simulink model "simon_loop_unrolling_4"  (R2015b)
settings: Solver=FixedStepDiscrete  SolverMode=SingleTasking  StartTime=0.0  StopTime=5e-4  RelTol=1e-3
undefined symbols (not defined in the file): a, b
libraries: shlslibv1 x190
settings Model: synDspstartup=OK  Creator=pgali  LastModifiedBy=sjparekh
settings DataIOCC: SaveOutput=off  SignalLogging=off  SaveTime=off
settings OptimizationCC: DefaultParameterBehavior=Inlined
settings DebuggingCC: AlgebraicLoopMsg=error  InheritedTsInSrcMsg=none

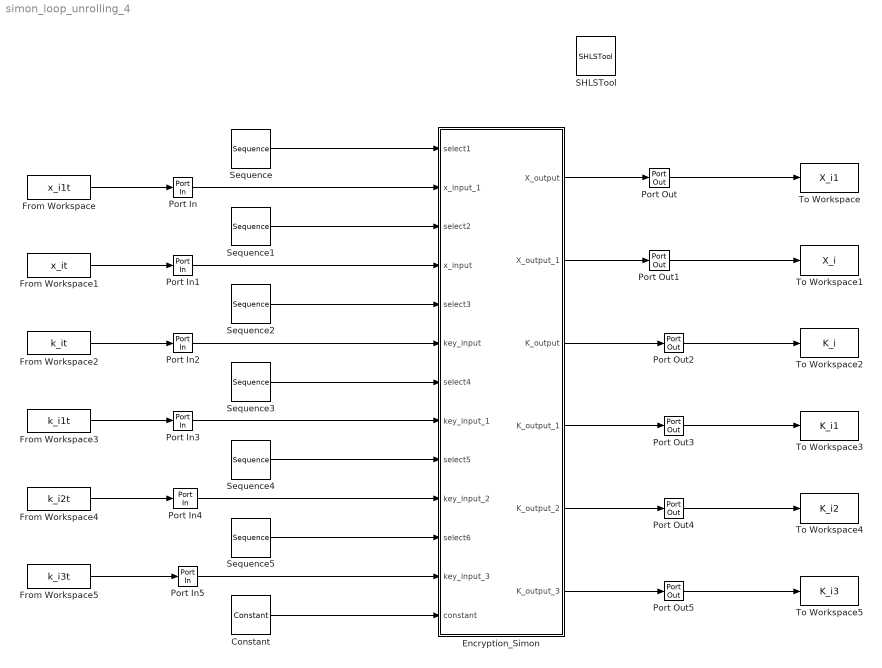
== system simon_loop_unrolling_4 ==
  Constant : shlslibv1/Sources/Constant  syn_cst_val=65532  syn_cst_format=Automatic  syn_cst_wl=1  syn_cst_fl=0  syn_cst_dt=unsigned  syn_cst_rnd=on  syn_cst_st=1/748e6  synBlockType=primitive  synLatency=0  synBlockId=15
  "Encryption_Simon " : Subsystem
  From Workspace : FromWorkspace  VariableName=x_i1t  SampleTime=0
  From Workspace1 : FromWorkspace  VariableName=x_it  SampleTime=0
  From Workspace2 : FromWorkspace  VariableName=k_it  SampleTime=0
  From Workspace3 : FromWorkspace  VariableName=k_i1t  SampleTime=0
  From Workspace4 : FromWorkspace  VariableName=k_i2t  SampleTime=0
  From Workspace5 : FromWorkspace  VariableName=k_i3t  SampleTime=0
  Port In{,1..5} (6 alike) : shlslibv1/Ports & Subsystems/Port In  syn_out_wl=16  syn_out_fl=0  syn_out_dt=unsigned  syn_out_st=1/748e6  syn_capture=off  syn_register=on  syn_out_sat=off  syn_out_rnd=on  synBlockType=port  synLatency=1  synBlockId=0
  Port Out{,1..5} (6 alike) : shlslibv1/Ports & Subsystems/Port Out  syn_capture=off  syn_register=on  synBlockType=port  synLatency=1  synBlockId=1
  SHLSTool : shlslibv1/SHLSTool  synBlockType=tool  syn_dsp_mode=FPGA
  Sequence{,1..5} (6 alike) : shlslibv1/Sources/Sequence  syn_seq_vec=[0 0 0 0 1 1 1 1 1 1 1 1 1 1 1 1 1 1 1 1 1 1 1 1 1 1 1 1 1 1 1 1]  syn_seq_wl=1  syn_seq_fl=0  syn_seq_dt=unsigned  syn_rst_port=off  syn_en_port=off  syn_seq_st=1/748e6  synBlockType=custom  synLatency=1
  To Workspace : ToWorkspace  VariableName=X_i1  SaveFormat=Structure With Time  SampleTime=-1
  To Workspace1 : ToWorkspace  VariableName=X_i  SaveFormat=Structure With Time  SampleTime=-1
  To Workspace2 : ToWorkspace  VariableName=K_i  SaveFormat=Structure With Time  SampleTime=-1
  To Workspace3 : ToWorkspace  VariableName=K_i1  SaveFormat=Structure With Time  SampleTime=-1
  To Workspace4 : ToWorkspace  VariableName=K_i2  SaveFormat=Structure With Time  SampleTime=-1
  To Workspace5 : ToWorkspace  VariableName=K_i3  SaveFormat=Structure With Time  SampleTime=-1
  wires:
  From Workspace1/1 -> Port In1/1
  From Workspace2/1 -> Port In2/1
  "Encryption_Simon "/1(X_output) -> Port Out/1
  "Encryption_Simon "/2(X_output_1) -> Port Out1/1
  "Encryption_Simon "/3(K_output) -> Port Out2/1
  "Encryption_Simon "/4(K_output_1) -> Port Out3/1
  "Encryption_Simon "/5(K_output_2) -> Port Out4/1
  "Encryption_Simon "/6(K_output_3) -> Port Out5/1
  From Workspace/1 -> Port In/1
  Constant/1 -> "Encryption_Simon "/13(constant)
  From Workspace3/1 -> Port In3/1
  From Workspace4/1 -> Port In4/1
  From Workspace5/1 -> Port In5/1
  Port In/1 -> "Encryption_Simon "/2(x_input_1)
  Port In1/1 -> "Encryption_Simon "/4(x_input)
  Port In2/1 -> "Encryption_Simon "/6(key_input)
  Port In3/1 -> "Encryption_Simon "/8(key_input_1)
  Port In4/1 -> "Encryption_Simon "/10(key_input_2)
  Port In5/1 -> "Encryption_Simon "/12(key_input_3)
  Port Out/1 -> To Workspace/1
  Port Out1/1 -> To Workspace1/1
  Port Out3/1 -> To Workspace3/1
  Port Out4/1 -> To Workspace4/1
  Port Out5/1 -> To Workspace5/1
  Port Out2/1 -> To Workspace2/1
  Sequence/1 -> "Encryption_Simon "/1(select1)
  Sequence1/1 -> "Encryption_Simon "/3(select2)
  Sequence2/1 -> "Encryption_Simon "/5(select3)
  Sequence3/1 -> "Encryption_Simon "/7(select4)
  Sequence4/1 -> "Encryption_Simon "/9(select5)
  Sequence5/1 -> "Encryption_Simon "/11(select6)

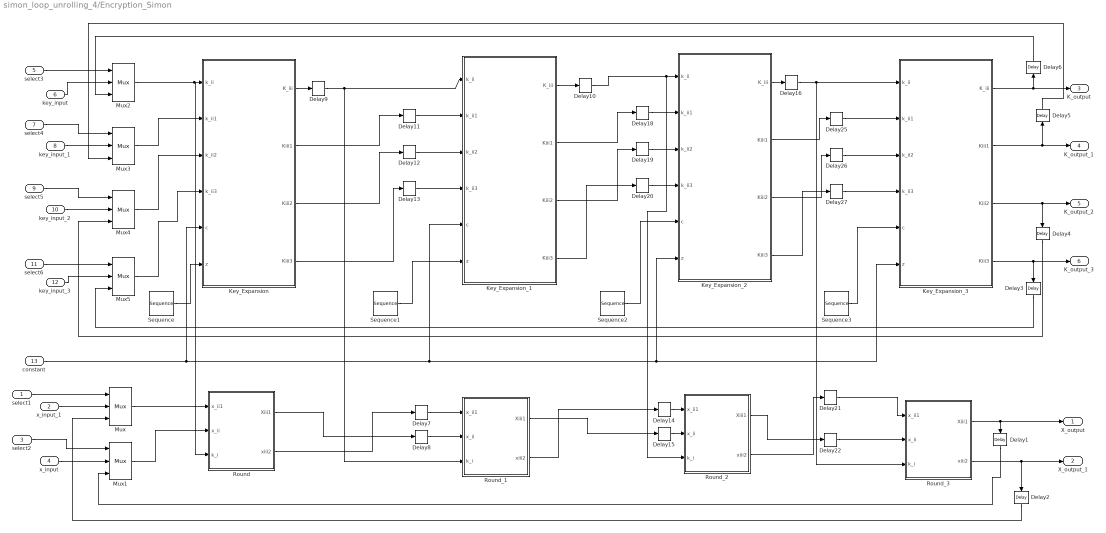
== system simon_loop_unrolling_4/Encryption_Simon  ==
  select1 : Inport
  x_input_1 : Inport  Port=2
  select2 : Inport  Port=3
  x_input : Inport  Port=4
  select3 : Inport  Port=5
  key_input : Inport  Port=6
  select4 : Inport  Port=7
  key_input_1 : Inport  Port=8
  select5 : Inport  Port=9
  key_input_2 : Inport  Port=10
  select6 : Inport  Port=11
  key_input_3 : Inport  Port=12
  constant : Inport  Port=13
  Delay{1..16,18..22,25..27} (24 alike) : shlslibv1/Memories/Delay  syn_delay_val=1  synBlockType=primitive  synLatency=1  synBlockId=104
  Key_Expansion : Subsystem
  Key_Expansion_1 : Subsystem
  Key_Expansion_2 : Subsystem
  Key_Expansion_3 : Subsystem
  Mux{,1..5} (6 alike) : shlslibv1/Signal Operations/Mux  syn_in_nb=2  syn_out_f=Full Precision  syn_out_wl=16  syn_out_fl=8  syn_out_dt=signed  syn_en_se=off  synBlockType=primitive  synLatency=0  synBlockId=16
  Round : Subsystem
  Round_1 : Subsystem
  Round_2 : Subsystem
  Round_3 : Subsystem
  Sequence : shlslibv1/Sources/Sequence  syn_seq_vec=[1 1 1 1 1 1 1 1 0 0 0 0 0 0 0 0 0 0 0 0 0 0 0 0 1 1 1 1 1 1 1 1]  syn_seq_wl=16  syn_seq_fl=0  syn_seq_dt=unsigned  syn_rst_port=off  syn_en_port=off  syn_seq_st=-1  synBlockType=custom  synLatency=1
  Sequence1 : shlslibv1/Sources/Sequence  syn_seq_vec=[0 1 1 1 1 0 0 0 0 0 0 0 0 1 1 1 1 1 1 1 1 0 0 0 0 1 1 1 1 1 1 1]  syn_seq_wl=16  syn_seq_fl=0  syn_seq_dt=unsigned  syn_rst_port=off  syn_en_port=off  syn_seq_st=-1  synBlockType=custom  synLatency=1
  Sequence2 : shlslibv1/Sources/Sequence  syn_seq_vec=[0 0 1 1 1 1 1 1 1 1 1 1 1 1 0 0 0 0 1 1 1 1 0 0 0 0 0 0 0 0 0 0]  syn_seq_wl=16  syn_seq_fl=0  syn_seq_dt=unsigned  syn_rst_port=off  syn_en_port=off  syn_seq_st=-1  synBlockType=custom  synLatency=1
  Sequence3 : shlslibv1/Sources/Sequence  syn_seq_vec=[0 0 0 1 1 1 1 0 0 0 0 0 0 0 0 1 1 1 1 0 0 0 0 1 1 1 1 0 0 0 0 0]  syn_seq_wl=16  syn_seq_fl=0  syn_seq_dt=unsigned  syn_rst_port=off  syn_en_port=off  syn_seq_st=-1  synBlockType=custom  synLatency=1
  X_output : Outport
  X_output_1 : Outport  Port=2
  K_output : Outport  Port=3
  K_output_1 : Outport  Port=4
  K_output_2 : Outport  Port=5
  K_output_3 : Outport  Port=6
  wires:
  select1/1 -> Mux/1
  x_input_1/1 -> Mux/2
  select2/1 -> Mux1/1
  x_input/1 -> Mux1/2
  select3/1 -> Mux2/1
  select4/1 -> Mux3/1
  key_input_1/1 -> Mux3/2
  select5/1 -> Mux4/1
  key_input_2/1 -> Mux4/2
  select6/1 -> Mux5/1
  key_input_3/1 -> Mux5/2
  Key_Expansion/2(Kiii1) -> Delay11/1
  Key_Expansion/3(Kiii2) -> Delay12/1
  Key_Expansion/4(Kiii3) -> Delay13/1
  constant/1 -> Key_Expansion_1/5(c), Key_Expansion_3/6(z), Key_Expansion_2/6(z), Key_Expansion/5(c)
  key_input/1 -> Mux2/2
  Mux/1 -> Round/1(" x_ii1")
  Mux1/1 -> Round/2(x_ii)
  Mux2/1 -> Round/3(k_i), Key_Expansion/1(k_ii)
  Mux3/1 -> Key_Expansion/2(k_ii1)
  Mux4/1 -> Key_Expansion/3(k_ii2)
  Mux5/1 -> Key_Expansion/4(k_ii3)
  Sequence/1 -> Key_Expansion/6(z)
  Round/2(xiii2) -> Delay7/1
  Round/1(Xiii1) -> Delay8/1
  Round_1/1(Xiii1) -> Delay15/1
  Round_1/2(xiii2) -> Delay14/1
  Key_Expansion_1/2(Kiii1) -> Delay18/1
  Key_Expansion_1/3(Kiii2) -> Delay19/1
  Key_Expansion_1/4(Kiii3) -> Delay20/1
  Round_2/1(Xiii1) -> Delay22/1
  Round_2/2(xiii2) -> Delay21/1
  Key_Expansion_2/2(Kiii1) -> Delay25/1
  Key_Expansion_2/3(Kiii2) -> Delay26/1
  Key_Expansion_2/4(Kiii3) -> Delay27/1
  Round_3/2(xiii2) -> X_output_1/1, Delay2/1
  Round_3/1(Xiii1) -> Delay1/1, X_output/1
  Key_Expansion_3/1(K_iii) -> Delay6/1, K_output/1
  Key_Expansion_3/2(Kiii1) -> Delay5/1, K_output_1/1
  Key_Expansion_3/3(Kiii2) -> Delay4/1, K_output_2/1
  Key_Expansion_3/4(Kiii3) -> Delay3/1, K_output_3/1
  Delay1/1 -> Mux1/3
  Delay2/1 -> Mux/3
  Delay3/1 -> Mux5/3
  Delay4/1 -> Mux4/3
  Delay5/1 -> Mux3/3
  Delay6/1 -> Mux2/3
  Delay7/1 -> Round_1/1(" x_ii1")
  Delay8/1 -> Round_1/2(x_ii)
  Key_Expansion/1(K_iii) -> Delay9/1
  Delay11/1 -> Key_Expansion_1/2(k_ii1)
  Delay12/1 -> Key_Expansion_1/3(k_ii2)
  Delay13/1 -> Key_Expansion_1/4(k_ii3)
  Delay14/1 -> Round_2/1(" x_ii1")
  Delay15/1 -> Round_2/2(x_ii)
  Key_Expansion_1/1(K_iii) -> Delay10/1
  Delay18/1 -> Key_Expansion_2/2(k_ii1)
  Delay19/1 -> Key_Expansion_2/3(k_ii2)
  Delay20/1 -> Key_Expansion_2/4(k_ii3)
  Delay21/1 -> Round_3/1(" x_ii1")
  Delay22/1 -> Round_3/2(x_ii)
  Key_Expansion_2/1(K_iii) -> Delay16/1
  Delay25/1 -> Key_Expansion_3/2(k_ii1)
  Delay26/1 -> Key_Expansion_3/3(k_ii2)
  Delay27/1 -> Key_Expansion_3/4(k_ii3)
  Delay9/1 -> Key_Expansion_1/1(k_ii), Round_1/3(k_i)
  Delay10/1 -> Key_Expansion_2/1(k_ii), Round_2/3(k_i)
  Delay16/1 -> Key_Expansion_3/1(k_ii), Round_3/3(k_i)
  Sequence1/1 -> Key_Expansion_1/6(z)
  Sequence2/1 -> Key_Expansion_2/5(c)
  Sequence3/1 -> Key_Expansion_3/5(c)

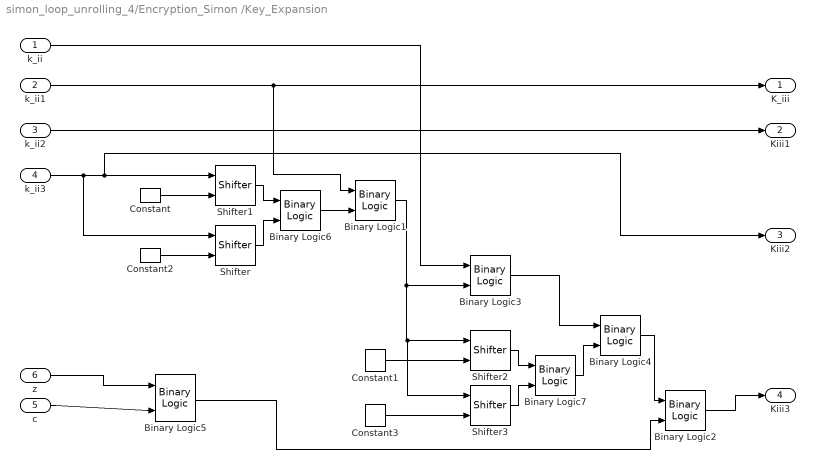
== system simon_loop_unrolling_4/Encryption_Simon /Key_Expansion ==
  k_ii : Inport
  k_ii1 : Inport  Port=2
  k_ii2 : Inport  Port=3
  k_ii3 : Inport  Port=4
  c : Inport  Port=5
  z : Inport  Port=6
  Binary Logic{1..5} (5 alike) : shlslibv1/Math Functions/Binary Logic  syn_binlog_exp=a^b  synBlockType=primitive  synLatency=0  synBlockId=13
  Binary Logic6 : shlslibv1/Math Functions/Binary Logic  syn_binlog_exp=a|b  synBlockType=primitive  synLatency=0  synBlockId=13
  Binary Logic7 : shlslibv1/Math Functions/Binary Logic  syn_binlog_exp=a|b  synBlockType=primitive  synLatency=0  synBlockId=13
  Constant : shlslibv1/Sources/Constant  syn_cst_val=3  syn_cst_format=Specify  syn_cst_wl=4  syn_cst_fl=0  syn_cst_dt=unsigned  syn_cst_rnd=on  syn_cst_st=-1  synBlockType=primitive  synLatency=0  synBlockId=15
  Constant1 : shlslibv1/Sources/Constant  syn_cst_val=1  syn_cst_format=Specify  syn_cst_wl=4  syn_cst_fl=0  syn_cst_dt=unsigned  syn_cst_rnd=on  syn_cst_st=-1  synBlockType=primitive  synLatency=0  synBlockId=15
  Constant2 : shlslibv1/Sources/Constant  syn_cst_val=13  syn_cst_format=Specify  syn_cst_wl=4  syn_cst_fl=0  syn_cst_dt=unsigned  syn_cst_rnd=on  syn_cst_st=-1  synBlockType=primitive  synLatency=0  synBlockId=15
  Constant3 : shlslibv1/Sources/Constant  syn_cst_val=15  syn_cst_format=Specify  syn_cst_wl=4  syn_cst_fl=0  syn_cst_dt=unsigned  syn_cst_rnd=on  syn_cst_st=-1  synBlockType=primitive  synLatency=0  synBlockId=15
  Shifter : shlslibv1/Math Functions/Shifter  syn_shifter_opr=<<  syn_out_f=Automatic  syn_out_wl=16  syn_out_fl=8  syn_out_dt=signed  synBlockType=primitive  synLatency=0  synBlockId=12
  Shifter1 : shlslibv1/Math Functions/Shifter  syn_shifter_opr=>>  syn_out_f=Automatic  syn_out_wl=16  syn_out_fl=8  syn_out_dt=signed  synBlockType=primitive  synLatency=0  synBlockId=12
  Shifter2 : shlslibv1/Math Functions/Shifter  syn_shifter_opr=>>  syn_out_f=Automatic  syn_out_wl=16  syn_out_fl=8  syn_out_dt=signed  synBlockType=primitive  synLatency=0  synBlockId=12
  Shifter3 : shlslibv1/Math Functions/Shifter  syn_shifter_opr=<<  syn_out_f=Automatic  syn_out_wl=16  syn_out_fl=8  syn_out_dt=signed  synBlockType=primitive  synLatency=0  synBlockId=12
  K_iii : Outport
  Kiii1 : Outport  Port=2
  Kiii2 : Outport  Port=3
  Kiii3 : Outport  Port=4
  wires:
  Binary Logic1/1 -> Shifter3/1, Shifter2/1, Binary Logic3/2
  Constant/1 -> Shifter1/2
  Constant1/1 -> Shifter2/2
  Binary Logic2/1 -> Kiii3/1
  Binary Logic4/1 -> Binary Logic2/1
  k_ii/1 -> Binary Logic3/1
  k_ii1/1 -> K_iii/1, Binary Logic1/1
  z/1 -> Binary Logic5/1
  c/1 -> Binary Logic5/2
  k_ii2/1 -> Kiii1/1
  k_ii3/1 -> Shifter/1, Shifter1/1, Kiii2/1
  Binary Logic3/1 -> Binary Logic4/1
  Binary Logic5/1 -> Binary Logic2/2
  Constant2/1 -> Shifter/2
  Shifter1/1 -> Binary Logic6/1
  Shifter/1 -> Binary Logic6/2
  Binary Logic6/1 -> Binary Logic1/2
  Constant3/1 -> Shifter3/2
  Shifter2/1 -> Binary Logic7/1
  Shifter3/1 -> Binary Logic7/2
  Binary Logic7/1 -> Binary Logic4/2

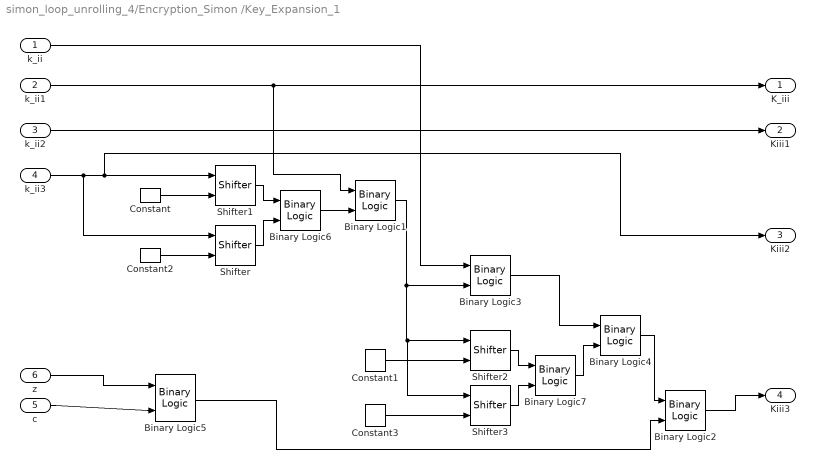
== system simon_loop_unrolling_4/Encryption_Simon /Key_Expansion_1 ==
  k_ii : Inport
  k_ii1 : Inport  Port=2
  k_ii2 : Inport  Port=3
  k_ii3 : Inport  Port=4
  c : Inport  Port=5
  z : Inport  Port=6
  Binary Logic{1..5} (5 alike) : shlslibv1/Math Functions/Binary Logic  syn_binlog_exp=a^b  synBlockType=primitive  synLatency=0  synBlockId=13
  Binary Logic6 : shlslibv1/Math Functions/Binary Logic  syn_binlog_exp=a|b  synBlockType=primitive  synLatency=0  synBlockId=13
  Binary Logic7 : shlslibv1/Math Functions/Binary Logic  syn_binlog_exp=a|b  synBlockType=primitive  synLatency=0  synBlockId=13
  Constant : shlslibv1/Sources/Constant  syn_cst_val=3  syn_cst_format=Specify  syn_cst_wl=4  syn_cst_fl=0  syn_cst_dt=unsigned  syn_cst_rnd=on  syn_cst_st=-1  synBlockType=primitive  synLatency=0  synBlockId=15
  Constant1 : shlslibv1/Sources/Constant  syn_cst_val=1  syn_cst_format=Specify  syn_cst_wl=4  syn_cst_fl=0  syn_cst_dt=unsigned  syn_cst_rnd=on  syn_cst_st=-1  synBlockType=primitive  synLatency=0  synBlockId=15
  Constant2 : shlslibv1/Sources/Constant  syn_cst_val=13  syn_cst_format=Specify  syn_cst_wl=4  syn_cst_fl=0  syn_cst_dt=unsigned  syn_cst_rnd=on  syn_cst_st=-1  synBlockType=primitive  synLatency=0  synBlockId=15
  Constant3 : shlslibv1/Sources/Constant  syn_cst_val=15  syn_cst_format=Specify  syn_cst_wl=4  syn_cst_fl=0  syn_cst_dt=unsigned  syn_cst_rnd=on  syn_cst_st=-1  synBlockType=primitive  synLatency=0  synBlockId=15
  Shifter : shlslibv1/Math Functions/Shifter  syn_shifter_opr=<<  syn_out_f=Automatic  syn_out_wl=16  syn_out_fl=8  syn_out_dt=signed  synBlockType=primitive  synLatency=0  synBlockId=12
  Shifter1 : shlslibv1/Math Functions/Shifter  syn_shifter_opr=>>  syn_out_f=Automatic  syn_out_wl=16  syn_out_fl=8  syn_out_dt=signed  synBlockType=primitive  synLatency=0  synBlockId=12
  Shifter2 : shlslibv1/Math Functions/Shifter  syn_shifter_opr=>>  syn_out_f=Automatic  syn_out_wl=16  syn_out_fl=8  syn_out_dt=signed  synBlockType=primitive  synLatency=0  synBlockId=12
  Shifter3 : shlslibv1/Math Functions/Shifter  syn_shifter_opr=<<  syn_out_f=Automatic  syn_out_wl=16  syn_out_fl=8  syn_out_dt=signed  synBlockType=primitive  synLatency=0  synBlockId=12
  K_iii : Outport
  Kiii1 : Outport  Port=2
  Kiii2 : Outport  Port=3
  Kiii3 : Outport  Port=4
  wires:
  Binary Logic1/1 -> Shifter3/1, Shifter2/1, Binary Logic3/2
  Constant/1 -> Shifter1/2
  Constant1/1 -> Shifter2/2
  Binary Logic2/1 -> Kiii3/1
  Binary Logic4/1 -> Binary Logic2/1
  k_ii/1 -> Binary Logic3/1
  k_ii1/1 -> K_iii/1, Binary Logic1/1
  z/1 -> Binary Logic5/1
  c/1 -> Binary Logic5/2
  k_ii2/1 -> Kiii1/1
  k_ii3/1 -> Shifter/1, Shifter1/1, Kiii2/1
  Binary Logic3/1 -> Binary Logic4/1
  Binary Logic5/1 -> Binary Logic2/2
  Constant2/1 -> Shifter/2
  Shifter1/1 -> Binary Logic6/1
  Shifter/1 -> Binary Logic6/2
  Binary Logic6/1 -> Binary Logic1/2
  Constant3/1 -> Shifter3/2
  Shifter2/1 -> Binary Logic7/1
  Shifter3/1 -> Binary Logic7/2
  Binary Logic7/1 -> Binary Logic4/2

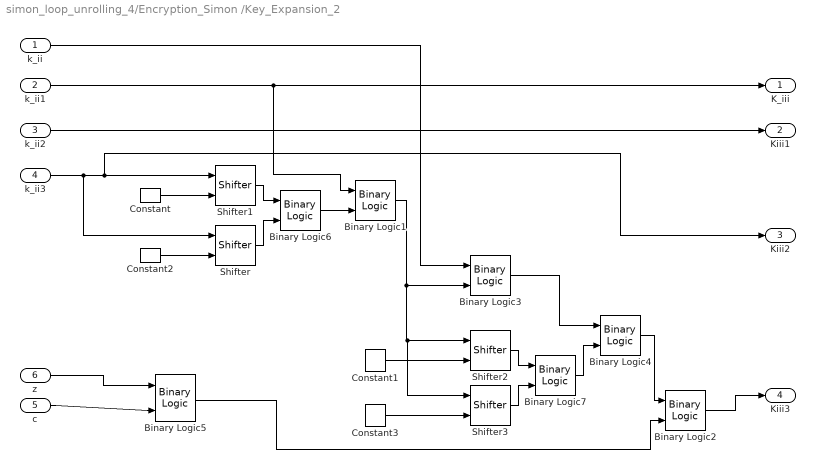
== system simon_loop_unrolling_4/Encryption_Simon /Key_Expansion_2 ==
  k_ii : Inport
  k_ii1 : Inport  Port=2
  k_ii2 : Inport  Port=3
  k_ii3 : Inport  Port=4
  c : Inport  Port=5
  z : Inport  Port=6
  Binary Logic{1..5} (5 alike) : shlslibv1/Math Functions/Binary Logic  syn_binlog_exp=a^b  synBlockType=primitive  synLatency=0  synBlockId=13
  Binary Logic6 : shlslibv1/Math Functions/Binary Logic  syn_binlog_exp=a|b  synBlockType=primitive  synLatency=0  synBlockId=13
  Binary Logic7 : shlslibv1/Math Functions/Binary Logic  syn_binlog_exp=a|b  synBlockType=primitive  synLatency=0  synBlockId=13
  Constant : shlslibv1/Sources/Constant  syn_cst_val=3  syn_cst_format=Specify  syn_cst_wl=4  syn_cst_fl=0  syn_cst_dt=unsigned  syn_cst_rnd=on  syn_cst_st=-1  synBlockType=primitive  synLatency=0  synBlockId=15
  Constant1 : shlslibv1/Sources/Constant  syn_cst_val=1  syn_cst_format=Specify  syn_cst_wl=4  syn_cst_fl=0  syn_cst_dt=unsigned  syn_cst_rnd=on  syn_cst_st=-1  synBlockType=primitive  synLatency=0  synBlockId=15
  Constant2 : shlslibv1/Sources/Constant  syn_cst_val=13  syn_cst_format=Specify  syn_cst_wl=4  syn_cst_fl=0  syn_cst_dt=unsigned  syn_cst_rnd=on  syn_cst_st=-1  synBlockType=primitive  synLatency=0  synBlockId=15
  Constant3 : shlslibv1/Sources/Constant  syn_cst_val=15  syn_cst_format=Specify  syn_cst_wl=4  syn_cst_fl=0  syn_cst_dt=unsigned  syn_cst_rnd=on  syn_cst_st=-1  synBlockType=primitive  synLatency=0  synBlockId=15
  Shifter : shlslibv1/Math Functions/Shifter  syn_shifter_opr=<<  syn_out_f=Automatic  syn_out_wl=16  syn_out_fl=8  syn_out_dt=signed  synBlockType=primitive  synLatency=0  synBlockId=12
  Shifter1 : shlslibv1/Math Functions/Shifter  syn_shifter_opr=>>  syn_out_f=Automatic  syn_out_wl=16  syn_out_fl=8  syn_out_dt=signed  synBlockType=primitive  synLatency=0  synBlockId=12
  Shifter2 : shlslibv1/Math Functions/Shifter  syn_shifter_opr=>>  syn_out_f=Automatic  syn_out_wl=16  syn_out_fl=8  syn_out_dt=signed  synBlockType=primitive  synLatency=0  synBlockId=12
  Shifter3 : shlslibv1/Math Functions/Shifter  syn_shifter_opr=<<  syn_out_f=Automatic  syn_out_wl=16  syn_out_fl=8  syn_out_dt=signed  synBlockType=primitive  synLatency=0  synBlockId=12
  K_iii : Outport
  Kiii1 : Outport  Port=2
  Kiii2 : Outport  Port=3
  Kiii3 : Outport  Port=4
  wires:
  Binary Logic1/1 -> Shifter3/1, Shifter2/1, Binary Logic3/2
  Constant/1 -> Shifter1/2
  Constant1/1 -> Shifter2/2
  Binary Logic2/1 -> Kiii3/1
  Binary Logic4/1 -> Binary Logic2/1
  k_ii/1 -> Binary Logic3/1
  k_ii1/1 -> K_iii/1, Binary Logic1/1
  z/1 -> Binary Logic5/1
  c/1 -> Binary Logic5/2
  k_ii2/1 -> Kiii1/1
  k_ii3/1 -> Shifter/1, Shifter1/1, Kiii2/1
  Binary Logic3/1 -> Binary Logic4/1
  Binary Logic5/1 -> Binary Logic2/2
  Constant2/1 -> Shifter/2
  Shifter1/1 -> Binary Logic6/1
  Shifter/1 -> Binary Logic6/2
  Binary Logic6/1 -> Binary Logic1/2
  Constant3/1 -> Shifter3/2
  Shifter2/1 -> Binary Logic7/1
  Shifter3/1 -> Binary Logic7/2
  Binary Logic7/1 -> Binary Logic4/2

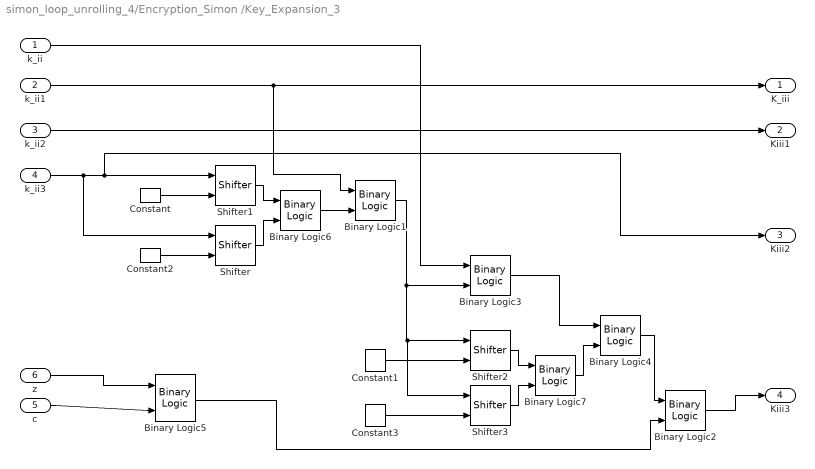
== system simon_loop_unrolling_4/Encryption_Simon /Key_Expansion_3 ==
  k_ii : Inport
  k_ii1 : Inport  Port=2
  k_ii2 : Inport  Port=3
  k_ii3 : Inport  Port=4
  c : Inport  Port=5
  z : Inport  Port=6
  Binary Logic{1..5} (5 alike) : shlslibv1/Math Functions/Binary Logic  syn_binlog_exp=a^b  synBlockType=primitive  synLatency=0  synBlockId=13
  Binary Logic6 : shlslibv1/Math Functions/Binary Logic  syn_binlog_exp=a|b  synBlockType=primitive  synLatency=0  synBlockId=13
  Binary Logic7 : shlslibv1/Math Functions/Binary Logic  syn_binlog_exp=a|b  synBlockType=primitive  synLatency=0  synBlockId=13
  Constant : shlslibv1/Sources/Constant  syn_cst_val=3  syn_cst_format=Specify  syn_cst_wl=4  syn_cst_fl=0  syn_cst_dt=unsigned  syn_cst_rnd=on  syn_cst_st=-1  synBlockType=primitive  synLatency=0  synBlockId=15
  Constant1 : shlslibv1/Sources/Constant  syn_cst_val=1  syn_cst_format=Specify  syn_cst_wl=4  syn_cst_fl=0  syn_cst_dt=unsigned  syn_cst_rnd=on  syn_cst_st=-1  synBlockType=primitive  synLatency=0  synBlockId=15
  Constant2 : shlslibv1/Sources/Constant  syn_cst_val=13  syn_cst_format=Specify  syn_cst_wl=4  syn_cst_fl=0  syn_cst_dt=unsigned  syn_cst_rnd=on  syn_cst_st=-1  synBlockType=primitive  synLatency=0  synBlockId=15
  Constant3 : shlslibv1/Sources/Constant  syn_cst_val=15  syn_cst_format=Specify  syn_cst_wl=4  syn_cst_fl=0  syn_cst_dt=unsigned  syn_cst_rnd=on  syn_cst_st=-1  synBlockType=primitive  synLatency=0  synBlockId=15
  Shifter : shlslibv1/Math Functions/Shifter  syn_shifter_opr=<<  syn_out_f=Automatic  syn_out_wl=16  syn_out_fl=8  syn_out_dt=signed  synBlockType=primitive  synLatency=0  synBlockId=12
  Shifter1 : shlslibv1/Math Functions/Shifter  syn_shifter_opr=>>  syn_out_f=Automatic  syn_out_wl=16  syn_out_fl=8  syn_out_dt=signed  synBlockType=primitive  synLatency=0  synBlockId=12
  Shifter2 : shlslibv1/Math Functions/Shifter  syn_shifter_opr=>>  syn_out_f=Automatic  syn_out_wl=16  syn_out_fl=8  syn_out_dt=signed  synBlockType=primitive  synLatency=0  synBlockId=12
  Shifter3 : shlslibv1/Math Functions/Shifter  syn_shifter_opr=<<  syn_out_f=Automatic  syn_out_wl=16  syn_out_fl=8  syn_out_dt=signed  synBlockType=primitive  synLatency=0  synBlockId=12
  K_iii : Outport
  Kiii1 : Outport  Port=2
  Kiii2 : Outport  Port=3
  Kiii3 : Outport  Port=4
  wires:
  Binary Logic1/1 -> Shifter3/1, Shifter2/1, Binary Logic3/2
  Constant/1 -> Shifter1/2
  Constant1/1 -> Shifter2/2
  Binary Logic2/1 -> Kiii3/1
  Binary Logic4/1 -> Binary Logic2/1
  k_ii/1 -> Binary Logic3/1
  k_ii1/1 -> K_iii/1, Binary Logic1/1
  z/1 -> Binary Logic5/1
  c/1 -> Binary Logic5/2
  k_ii2/1 -> Kiii1/1
  k_ii3/1 -> Shifter/1, Shifter1/1, Kiii2/1
  Binary Logic3/1 -> Binary Logic4/1
  Binary Logic5/1 -> Binary Logic2/2
  Constant2/1 -> Shifter/2
  Shifter1/1 -> Binary Logic6/1
  Shifter/1 -> Binary Logic6/2
  Binary Logic6/1 -> Binary Logic1/2
  Constant3/1 -> Shifter3/2
  Shifter2/1 -> Binary Logic7/1
  Shifter3/1 -> Binary Logic7/2
  Binary Logic7/1 -> Binary Logic4/2

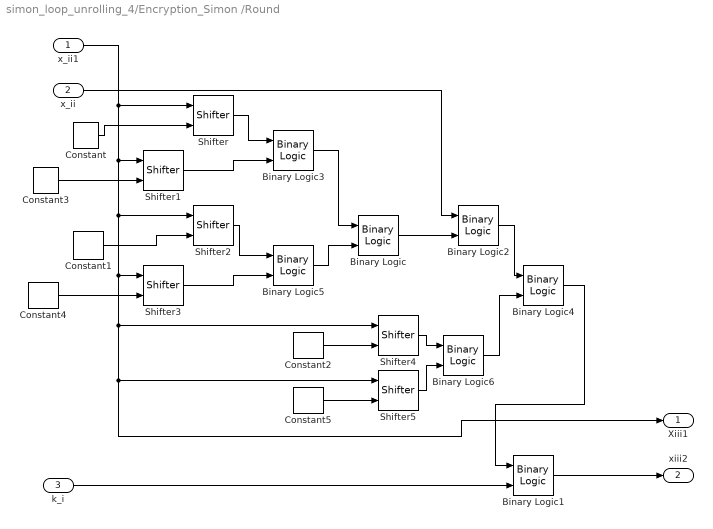
== system simon_loop_unrolling_4/Encryption_Simon /Round ==
  " x_ii1" : Inport  OutMin=[0]  OutMax=[0]
  x_ii : Inport  Port=2  OutMin=[0]  OutMax=[0]
  k_i : Inport  Port=3  OutMin=[0]  OutMax=[0]
  Binary Logic : shlslibv1/Math Functions/Binary Logic  syn_binlog_exp=a&b  synBlockType=primitive  synLatency=0  synBlockId=13
  Binary Logic1 : shlslibv1/Math Functions/Binary Logic  syn_binlog_exp=a^b  synBlockType=primitive  synLatency=0  synBlockId=13
  Binary Logic2 : shlslibv1/Math Functions/Binary Logic  syn_binlog_exp=a^b  synBlockType=primitive  synLatency=0  synBlockId=13
  Binary Logic3 : shlslibv1/Math Functions/Binary Logic  syn_binlog_exp=a|b  synBlockType=primitive  synLatency=0  synBlockId=13
  Binary Logic4 : shlslibv1/Math Functions/Binary Logic  syn_binlog_exp=a^b  synBlockType=primitive  synLatency=0  synBlockId=13
  Binary Logic5 : shlslibv1/Math Functions/Binary Logic  syn_binlog_exp=a|b  synBlockType=primitive  synLatency=0  synBlockId=13
  Binary Logic6 : shlslibv1/Math Functions/Binary Logic  syn_binlog_exp=a|b  synBlockType=primitive  synLatency=0  synBlockId=13
  Constant : shlslibv1/Sources/Constant  syn_cst_val=1  syn_cst_format=Specify  syn_cst_wl=4  syn_cst_fl=0  syn_cst_dt=unsigned  syn_cst_rnd=on  syn_cst_st=-1  synBlockType=primitive  synLatency=0  synBlockId=15
  Constant1 : shlslibv1/Sources/Constant  syn_cst_val=8  syn_cst_format=Specify  syn_cst_wl=4  syn_cst_fl=0  syn_cst_dt=unsigned  syn_cst_rnd=on  syn_cst_st=-1  synBlockType=primitive  synLatency=0  synBlockId=15
  Constant2 : shlslibv1/Sources/Constant  syn_cst_val=2  syn_cst_format=Specify  syn_cst_wl=4  syn_cst_fl=0  syn_cst_dt=unsigned  syn_cst_rnd=on  syn_cst_st=-1  synBlockType=primitive  synLatency=0  synBlockId=15
  Constant3 : shlslibv1/Sources/Constant  syn_cst_val=15  syn_cst_format=Specify  syn_cst_wl=4  syn_cst_fl=0  syn_cst_dt=unsigned  syn_cst_rnd=on  syn_cst_st=-1  synBlockType=primitive  synLatency=0  synBlockId=15
  Constant4 : shlslibv1/Sources/Constant  syn_cst_val=8  syn_cst_format=Specify  syn_cst_wl=4  syn_cst_fl=0  syn_cst_dt=unsigned  syn_cst_rnd=on  syn_cst_st=-1  synBlockType=primitive  synLatency=0  synBlockId=15
  Constant5 : shlslibv1/Sources/Constant  syn_cst_val=14  syn_cst_format=Specify  syn_cst_wl=4  syn_cst_fl=0  syn_cst_dt=unsigned  syn_cst_rnd=on  syn_cst_st=-1  synBlockType=primitive  synLatency=0  synBlockId=15
  Shifter : shlslibv1/Math Functions/Shifter  syn_shifter_opr=<<  syn_out_f=Automatic  syn_out_wl=16  syn_out_fl=8  syn_out_dt=signed  synBlockType=primitive  synLatency=0  synBlockId=12
  Shifter1 : shlslibv1/Math Functions/Shifter  syn_shifter_opr=>>  syn_out_f=Automatic  syn_out_wl=16  syn_out_fl=8  syn_out_dt=signed  synBlockType=primitive  synLatency=0  synBlockId=12
  Shifter2 : shlslibv1/Math Functions/Shifter  syn_shifter_opr=<<  syn_out_f=Automatic  syn_out_wl=16  syn_out_fl=8  syn_out_dt=signed  synBlockType=primitive  synLatency=0  synBlockId=12
  Shifter3 : shlslibv1/Math Functions/Shifter  syn_shifter_opr=>>  syn_out_f=Automatic  syn_out_wl=16  syn_out_fl=8  syn_out_dt=signed  synBlockType=primitive  synLatency=0  synBlockId=12
  Shifter4 : shlslibv1/Math Functions/Shifter  syn_shifter_opr=<<  syn_out_f=Automatic  syn_out_wl=16  syn_out_fl=8  syn_out_dt=signed  synBlockType=primitive  synLatency=0  synBlockId=12
  Shifter5 : shlslibv1/Math Functions/Shifter  syn_shifter_opr=>>  syn_out_f=Automatic  syn_out_wl=16  syn_out_fl=8  syn_out_dt=signed  synBlockType=primitive  synLatency=0  synBlockId=12
  Xiii1 : Outport
  xiii2 : Outport  Port=2
  wires:
  Binary Logic/1 -> Binary Logic2/2
  Binary Logic2/1 -> Binary Logic4/1
  Binary Logic4/1 -> Binary Logic1/1
  Constant/1 -> Shifter/2
  Constant1/1 -> Shifter2/2
  Binary Logic1/1 -> xiii2/1
  x_ii/1 -> Binary Logic2/1
  " x_ii1"/1 -> Shifter1/1, Shifter2/1, Shifter4/1, Xiii1/1, Shifter5/1, Shifter3/1, Shifter/1
  k_i/1 -> Binary Logic1/2
  Constant3/1 -> Shifter1/2
  Shifter/1 -> Binary Logic3/1
  Shifter1/1 -> Binary Logic3/2
  Binary Logic3/1 -> Binary Logic/1
  Constant4/1 -> Shifter3/2
  Shifter2/1 -> Binary Logic5/1
  Shifter3/1 -> Binary Logic5/2
  Binary Logic5/1 -> Binary Logic/2
  Constant2/1 -> Shifter4/2
  Shifter4/1 -> Binary Logic6/1
  Constant5/1 -> Shifter5/2
  Shifter5/1 -> Binary Logic6/2
  Binary Logic6/1 -> Binary Logic4/2

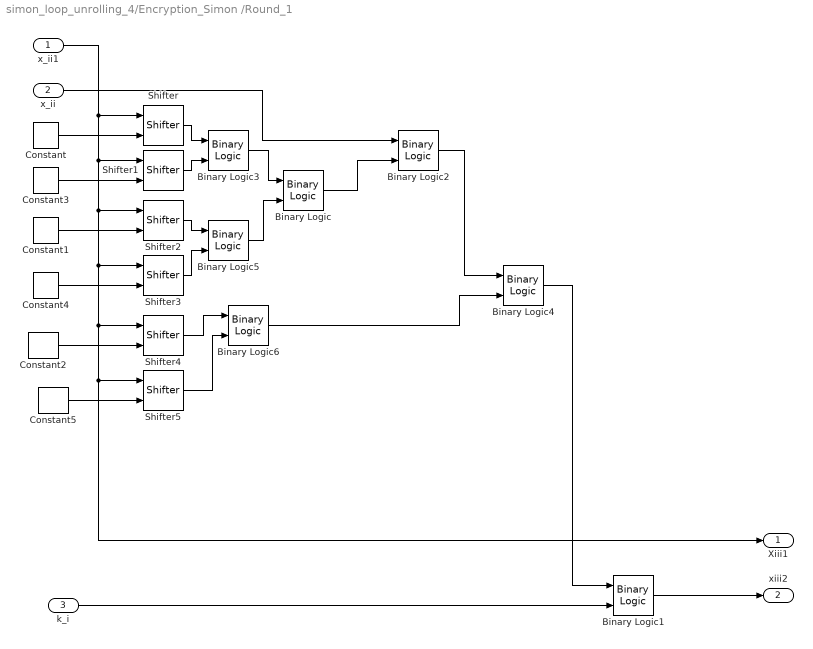
== system simon_loop_unrolling_4/Encryption_Simon /Round_1 ==
  " x_ii1" : Inport  OutMin=[0]  OutMax=[0]
  x_ii : Inport  Port=2  OutMin=[0]  OutMax=[0]
  k_i : Inport  Port=3  OutMin=[0]  OutMax=[0]
  Binary Logic : shlslibv1/Math Functions/Binary Logic  syn_binlog_exp=a&b  synBlockType=primitive  synLatency=0  synBlockId=13
  Binary Logic1 : shlslibv1/Math Functions/Binary Logic  syn_binlog_exp=a^b  synBlockType=primitive  synLatency=0  synBlockId=13
  Binary Logic2 : shlslibv1/Math Functions/Binary Logic  syn_binlog_exp=a^b  synBlockType=primitive  synLatency=0  synBlockId=13
  Binary Logic3 : shlslibv1/Math Functions/Binary Logic  syn_binlog_exp=a|b  synBlockType=primitive  synLatency=0  synBlockId=13
  Binary Logic4 : shlslibv1/Math Functions/Binary Logic  syn_binlog_exp=a^b  synBlockType=primitive  synLatency=0  synBlockId=13
  Binary Logic5 : shlslibv1/Math Functions/Binary Logic  syn_binlog_exp=a|b  synBlockType=primitive  synLatency=0  synBlockId=13
  Binary Logic6 : shlslibv1/Math Functions/Binary Logic  syn_binlog_exp=a|b  synBlockType=primitive  synLatency=0  synBlockId=13
  Constant : shlslibv1/Sources/Constant  syn_cst_val=1  syn_cst_format=Specify  syn_cst_wl=4  syn_cst_fl=0  syn_cst_dt=unsigned  syn_cst_rnd=on  syn_cst_st=-1  synBlockType=primitive  synLatency=0  synBlockId=15
  Constant1 : shlslibv1/Sources/Constant  syn_cst_val=8  syn_cst_format=Specify  syn_cst_wl=4  syn_cst_fl=0  syn_cst_dt=unsigned  syn_cst_rnd=on  syn_cst_st=-1  synBlockType=primitive  synLatency=0  synBlockId=15
  Constant2 : shlslibv1/Sources/Constant  syn_cst_val=2  syn_cst_format=Specify  syn_cst_wl=4  syn_cst_fl=0  syn_cst_dt=unsigned  syn_cst_rnd=on  syn_cst_st=-1  synBlockType=primitive  synLatency=0  synBlockId=15
  Constant3 : shlslibv1/Sources/Constant  syn_cst_val=15  syn_cst_format=Specify  syn_cst_wl=4  syn_cst_fl=0  syn_cst_dt=unsigned  syn_cst_rnd=on  syn_cst_st=-1  synBlockType=primitive  synLatency=0  synBlockId=15
  Constant4 : shlslibv1/Sources/Constant  syn_cst_val=8  syn_cst_format=Specify  syn_cst_wl=4  syn_cst_fl=0  syn_cst_dt=unsigned  syn_cst_rnd=on  syn_cst_st=-1  synBlockType=primitive  synLatency=0  synBlockId=15
  Constant5 : shlslibv1/Sources/Constant  syn_cst_val=14  syn_cst_format=Specify  syn_cst_wl=4  syn_cst_fl=0  syn_cst_dt=unsigned  syn_cst_rnd=on  syn_cst_st=-1  synBlockType=primitive  synLatency=0  synBlockId=15
  Shifter : shlslibv1/Math Functions/Shifter  syn_shifter_opr=<<  syn_out_f=Automatic  syn_out_wl=16  syn_out_fl=8  syn_out_dt=signed  synBlockType=primitive  synLatency=0  synBlockId=12
  Shifter1 : shlslibv1/Math Functions/Shifter  syn_shifter_opr=>>  syn_out_f=Automatic  syn_out_wl=16  syn_out_fl=8  syn_out_dt=signed  synBlockType=primitive  synLatency=0  synBlockId=12
  Shifter2 : shlslibv1/Math Functions/Shifter  syn_shifter_opr=<<  syn_out_f=Automatic  syn_out_wl=16  syn_out_fl=8  syn_out_dt=signed  synBlockType=primitive  synLatency=0  synBlockId=12
  Shifter3 : shlslibv1/Math Functions/Shifter  syn_shifter_opr=>>  syn_out_f=Automatic  syn_out_wl=16  syn_out_fl=8  syn_out_dt=signed  synBlockType=primitive  synLatency=0  synBlockId=12
  Shifter4 : shlslibv1/Math Functions/Shifter  syn_shifter_opr=<<  syn_out_f=Automatic  syn_out_wl=16  syn_out_fl=8  syn_out_dt=signed  synBlockType=primitive  synLatency=0  synBlockId=12
  Shifter5 : shlslibv1/Math Functions/Shifter  syn_shifter_opr=>>  syn_out_f=Automatic  syn_out_wl=16  syn_out_fl=8  syn_out_dt=signed  synBlockType=primitive  synLatency=0  synBlockId=12
  Xiii1 : Outport
  xiii2 : Outport  Port=2
  wires:
  Binary Logic/1 -> Binary Logic2/2
  Binary Logic2/1 -> Binary Logic4/1
  Binary Logic4/1 -> Binary Logic1/1
  Constant/1 -> Shifter/2
  Constant1/1 -> Shifter2/2
  Binary Logic1/1 -> xiii2/1
  x_ii/1 -> Binary Logic2/1
  " x_ii1"/1 -> Shifter/1, Shifter1/1, Shifter2/1, Shifter3/1, Shifter4/1, Xiii1/1, Shifter5/1
  k_i/1 -> Binary Logic1/2
  Constant3/1 -> Shifter1/2
  Shifter/1 -> Binary Logic3/1
  Shifter1/1 -> Binary Logic3/2
  Binary Logic3/1 -> Binary Logic/1
  Constant4/1 -> Shifter3/2
  Shifter2/1 -> Binary Logic5/1
  Shifter3/1 -> Binary Logic5/2
  Binary Logic5/1 -> Binary Logic/2
  Constant2/1 -> Shifter4/2
  Shifter4/1 -> Binary Logic6/1
  Constant5/1 -> Shifter5/2
  Shifter5/1 -> Binary Logic6/2
  Binary Logic6/1 -> Binary Logic4/2

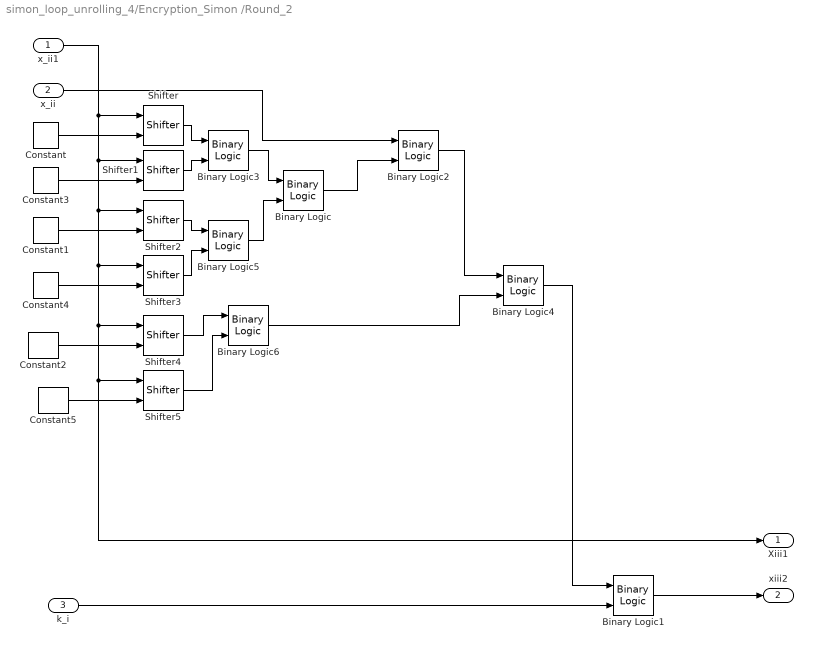
== system simon_loop_unrolling_4/Encryption_Simon /Round_2 ==
  " x_ii1" : Inport  OutMin=[0]  OutMax=[0]
  x_ii : Inport  Port=2  OutMin=[0]  OutMax=[0]
  k_i : Inport  Port=3  OutMin=[0]  OutMax=[0]
  Binary Logic : shlslibv1/Math Functions/Binary Logic  syn_binlog_exp=a&b  synBlockType=primitive  synLatency=0  synBlockId=13
  Binary Logic1 : shlslibv1/Math Functions/Binary Logic  syn_binlog_exp=a^b  synBlockType=primitive  synLatency=0  synBlockId=13
  Binary Logic2 : shlslibv1/Math Functions/Binary Logic  syn_binlog_exp=a^b  synBlockType=primitive  synLatency=0  synBlockId=13
  Binary Logic3 : shlslibv1/Math Functions/Binary Logic  syn_binlog_exp=a|b  synBlockType=primitive  synLatency=0  synBlockId=13
  Binary Logic4 : shlslibv1/Math Functions/Binary Logic  syn_binlog_exp=a^b  synBlockType=primitive  synLatency=0  synBlockId=13
  Binary Logic5 : shlslibv1/Math Functions/Binary Logic  syn_binlog_exp=a|b  synBlockType=primitive  synLatency=0  synBlockId=13
  Binary Logic6 : shlslibv1/Math Functions/Binary Logic  syn_binlog_exp=a|b  synBlockType=primitive  synLatency=0  synBlockId=13
  Constant : shlslibv1/Sources/Constant  syn_cst_val=1  syn_cst_format=Specify  syn_cst_wl=4  syn_cst_fl=0  syn_cst_dt=unsigned  syn_cst_rnd=on  syn_cst_st=-1  synBlockType=primitive  synLatency=0  synBlockId=15
  Constant1 : shlslibv1/Sources/Constant  syn_cst_val=8  syn_cst_format=Specify  syn_cst_wl=4  syn_cst_fl=0  syn_cst_dt=unsigned  syn_cst_rnd=on  syn_cst_st=-1  synBlockType=primitive  synLatency=0  synBlockId=15
  Constant2 : shlslibv1/Sources/Constant  syn_cst_val=2  syn_cst_format=Specify  syn_cst_wl=4  syn_cst_fl=0  syn_cst_dt=unsigned  syn_cst_rnd=on  syn_cst_st=-1  synBlockType=primitive  synLatency=0  synBlockId=15
  Constant3 : shlslibv1/Sources/Constant  syn_cst_val=15  syn_cst_format=Specify  syn_cst_wl=4  syn_cst_fl=0  syn_cst_dt=unsigned  syn_cst_rnd=on  syn_cst_st=-1  synBlockType=primitive  synLatency=0  synBlockId=15
  Constant4 : shlslibv1/Sources/Constant  syn_cst_val=8  syn_cst_format=Specify  syn_cst_wl=4  syn_cst_fl=0  syn_cst_dt=unsigned  syn_cst_rnd=on  syn_cst_st=-1  synBlockType=primitive  synLatency=0  synBlockId=15
  Constant5 : shlslibv1/Sources/Constant  syn_cst_val=14  syn_cst_format=Specify  syn_cst_wl=4  syn_cst_fl=0  syn_cst_dt=unsigned  syn_cst_rnd=on  syn_cst_st=-1  synBlockType=primitive  synLatency=0  synBlockId=15
  Shifter : shlslibv1/Math Functions/Shifter  syn_shifter_opr=<<  syn_out_f=Automatic  syn_out_wl=16  syn_out_fl=8  syn_out_dt=signed  synBlockType=primitive  synLatency=0  synBlockId=12
  Shifter1 : shlslibv1/Math Functions/Shifter  syn_shifter_opr=>>  syn_out_f=Automatic  syn_out_wl=16  syn_out_fl=8  syn_out_dt=signed  synBlockType=primitive  synLatency=0  synBlockId=12
  Shifter2 : shlslibv1/Math Functions/Shifter  syn_shifter_opr=<<  syn_out_f=Automatic  syn_out_wl=16  syn_out_fl=8  syn_out_dt=signed  synBlockType=primitive  synLatency=0  synBlockId=12
  Shifter3 : shlslibv1/Math Functions/Shifter  syn_shifter_opr=>>  syn_out_f=Automatic  syn_out_wl=16  syn_out_fl=8  syn_out_dt=signed  synBlockType=primitive  synLatency=0  synBlockId=12
  Shifter4 : shlslibv1/Math Functions/Shifter  syn_shifter_opr=<<  syn_out_f=Automatic  syn_out_wl=16  syn_out_fl=8  syn_out_dt=signed  synBlockType=primitive  synLatency=0  synBlockId=12
  Shifter5 : shlslibv1/Math Functions/Shifter  syn_shifter_opr=>>  syn_out_f=Automatic  syn_out_wl=16  syn_out_fl=8  syn_out_dt=signed  synBlockType=primitive  synLatency=0  synBlockId=12
  Xiii1 : Outport
  xiii2 : Outport  Port=2
  wires:
  Binary Logic/1 -> Binary Logic2/2
  Binary Logic2/1 -> Binary Logic4/1
  Binary Logic4/1 -> Binary Logic1/1
  Constant/1 -> Shifter/2
  Constant1/1 -> Shifter2/2
  Binary Logic1/1 -> xiii2/1
  x_ii/1 -> Binary Logic2/1
  " x_ii1"/1 -> Shifter/1, Shifter1/1, Shifter2/1, Shifter3/1, Shifter4/1, Xiii1/1, Shifter5/1
  k_i/1 -> Binary Logic1/2
  Constant3/1 -> Shifter1/2
  Shifter/1 -> Binary Logic3/1
  Shifter1/1 -> Binary Logic3/2
  Binary Logic3/1 -> Binary Logic/1
  Constant4/1 -> Shifter3/2
  Shifter2/1 -> Binary Logic5/1
  Shifter3/1 -> Binary Logic5/2
  Binary Logic5/1 -> Binary Logic/2
  Constant2/1 -> Shifter4/2
  Shifter4/1 -> Binary Logic6/1
  Constant5/1 -> Shifter5/2
  Shifter5/1 -> Binary Logic6/2
  Binary Logic6/1 -> Binary Logic4/2

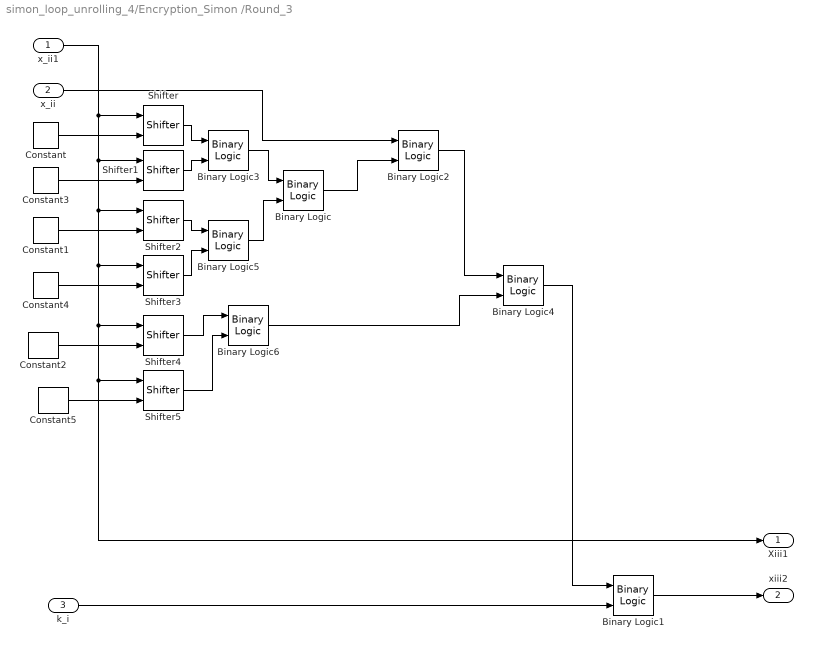
== system simon_loop_unrolling_4/Encryption_Simon /Round_3 ==
  " x_ii1" : Inport  OutMin=[0]  OutMax=[0]
  x_ii : Inport  Port=2  OutMin=[0]  OutMax=[0]
  k_i : Inport  Port=3  OutMin=[0]  OutMax=[0]
  Binary Logic : shlslibv1/Math Functions/Binary Logic  syn_binlog_exp=a&b  synBlockType=primitive  synLatency=0  synBlockId=13
  Binary Logic1 : shlslibv1/Math Functions/Binary Logic  syn_binlog_exp=a^b  synBlockType=primitive  synLatency=0  synBlockId=13
  Binary Logic2 : shlslibv1/Math Functions/Binary Logic  syn_binlog_exp=a^b  synBlockType=primitive  synLatency=0  synBlockId=13
  Binary Logic3 : shlslibv1/Math Functions/Binary Logic  syn_binlog_exp=a|b  synBlockType=primitive  synLatency=0  synBlockId=13
  Binary Logic4 : shlslibv1/Math Functions/Binary Logic  syn_binlog_exp=a^b  synBlockType=primitive  synLatency=0  synBlockId=13
  Binary Logic5 : shlslibv1/Math Functions/Binary Logic  syn_binlog_exp=a|b  synBlockType=primitive  synLatency=0  synBlockId=13
  Binary Logic6 : shlslibv1/Math Functions/Binary Logic  syn_binlog_exp=a|b  synBlockType=primitive  synLatency=0  synBlockId=13
  Constant : shlslibv1/Sources/Constant  syn_cst_val=1  syn_cst_format=Specify  syn_cst_wl=4  syn_cst_fl=0  syn_cst_dt=unsigned  syn_cst_rnd=on  syn_cst_st=-1  synBlockType=primitive  synLatency=0  synBlockId=15
  Constant1 : shlslibv1/Sources/Constant  syn_cst_val=8  syn_cst_format=Specify  syn_cst_wl=4  syn_cst_fl=0  syn_cst_dt=unsigned  syn_cst_rnd=on  syn_cst_st=-1  synBlockType=primitive  synLatency=0  synBlockId=15
  Constant2 : shlslibv1/Sources/Constant  syn_cst_val=2  syn_cst_format=Specify  syn_cst_wl=4  syn_cst_fl=0  syn_cst_dt=unsigned  syn_cst_rnd=on  syn_cst_st=-1  synBlockType=primitive  synLatency=0  synBlockId=15
  Constant3 : shlslibv1/Sources/Constant  syn_cst_val=15  syn_cst_format=Specify  syn_cst_wl=4  syn_cst_fl=0  syn_cst_dt=unsigned  syn_cst_rnd=on  syn_cst_st=-1  synBlockType=primitive  synLatency=0  synBlockId=15
  Constant4 : shlslibv1/Sources/Constant  syn_cst_val=8  syn_cst_format=Specify  syn_cst_wl=4  syn_cst_fl=0  syn_cst_dt=unsigned  syn_cst_rnd=on  syn_cst_st=-1  synBlockType=primitive  synLatency=0  synBlockId=15
  Constant5 : shlslibv1/Sources/Constant  syn_cst_val=14  syn_cst_format=Specify  syn_cst_wl=4  syn_cst_fl=0  syn_cst_dt=unsigned  syn_cst_rnd=on  syn_cst_st=-1  synBlockType=primitive  synLatency=0  synBlockId=15
  Shifter : shlslibv1/Math Functions/Shifter  syn_shifter_opr=<<  syn_out_f=Automatic  syn_out_wl=16  syn_out_fl=8  syn_out_dt=signed  synBlockType=primitive  synLatency=0  synBlockId=12
  Shifter1 : shlslibv1/Math Functions/Shifter  syn_shifter_opr=>>  syn_out_f=Automatic  syn_out_wl=16  syn_out_fl=8  syn_out_dt=signed  synBlockType=primitive  synLatency=0  synBlockId=12
  Shifter2 : shlslibv1/Math Functions/Shifter  syn_shifter_opr=<<  syn_out_f=Automatic  syn_out_wl=16  syn_out_fl=8  syn_out_dt=signed  synBlockType=primitive  synLatency=0  synBlockId=12
  Shifter3 : shlslibv1/Math Functions/Shifter  syn_shifter_opr=>>  syn_out_f=Automatic  syn_out_wl=16  syn_out_fl=8  syn_out_dt=signed  synBlockType=primitive  synLatency=0  synBlockId=12
  Shifter4 : shlslibv1/Math Functions/Shifter  syn_shifter_opr=<<  syn_out_f=Automatic  syn_out_wl=16  syn_out_fl=8  syn_out_dt=signed  synBlockType=primitive  synLatency=0  synBlockId=12
  Shifter5 : shlslibv1/Math Functions/Shifter  syn_shifter_opr=>>  syn_out_f=Automatic  syn_out_wl=16  syn_out_fl=8  syn_out_dt=signed  synBlockType=primitive  synLatency=0  synBlockId=12
  Xiii1 : Outport
  xiii2 : Outport  Port=2
  wires:
  Binary Logic/1 -> Binary Logic2/2
  Binary Logic2/1 -> Binary Logic4/1
  Binary Logic4/1 -> Binary Logic1/1
  Constant/1 -> Shifter/2
  Constant1/1 -> Shifter2/2
  Binary Logic1/1 -> xiii2/1
  x_ii/1 -> Binary Logic2/1
  " x_ii1"/1 -> Shifter/1, Shifter1/1, Shifter2/1, Shifter3/1, Shifter4/1, Xiii1/1, Shifter5/1
  k_i/1 -> Binary Logic1/2
  Constant3/1 -> Shifter1/2
  Shifter/1 -> Binary Logic3/1
  Shifter1/1 -> Binary Logic3/2
  Binary Logic3/1 -> Binary Logic/1
  Constant4/1 -> Shifter3/2
  Shifter2/1 -> Binary Logic5/1
  Shifter3/1 -> Binary Logic5/2
  Binary Logic5/1 -> Binary Logic/2
  Constant2/1 -> Shifter4/2
  Shifter4/1 -> Binary Logic6/1
  Constant5/1 -> Shifter5/2
  Shifter5/1 -> Binary Logic6/2
  Binary Logic6/1 -> Binary Logic4/2
